simulink model "OFDM"  (R2021a)
settings: Solver=VariableStepAuto  StartTime=0.0  StopTime=1000.0  RelTol=1e-3
InitFcn:
  | clear
  | %frequency
  | Fs = 20e6;
  | M =16;
  | 
  | fD=1;
  | Td=[0, 200, 300, 1300, 2700]*1e-09;
  | Pd=[0, -0.9, -3.9, -7.8, -13.9];
undefined symbols (not defined in the file or in its folder): doppler
libraries: commutil2 x2, dspxfrm3 x2, commdigbbndam3 x2, commrandsrc3 x1, commsink2 x1, commchan3 x1
settings Model: Creator=AJ  LastModifiedBy=AJ
settings SFSimCC: MATLABDynamicMemAllocThreshold=2147483647

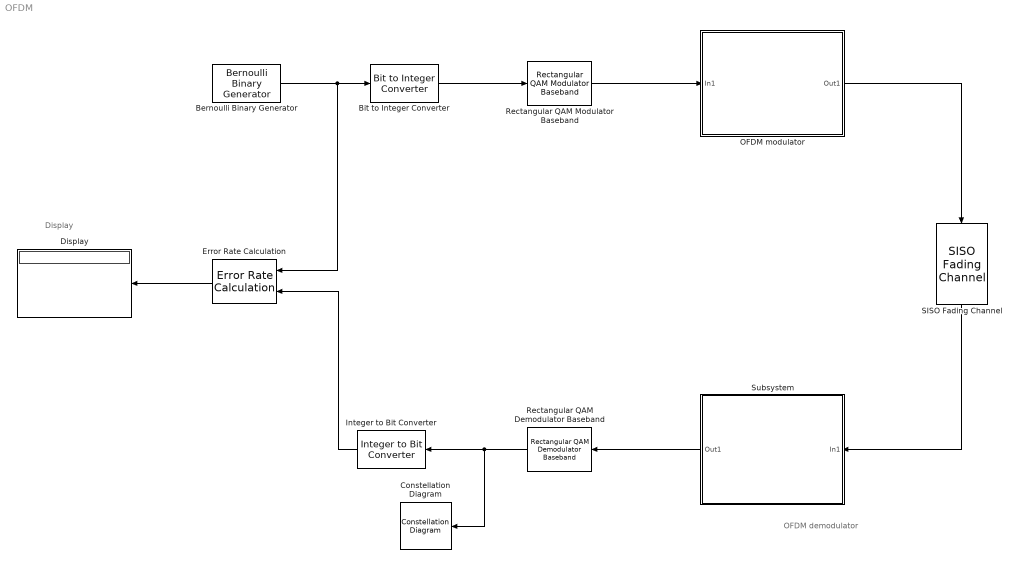
== system OFDM ==
  note: Display
  note: OFDM demodulator
  Bernoulli Binary Generator : commrandsrc3/Bernoulli Binary Generator  ProbabilityOfZero=0.5  SeedSource=Parameter  Seed=61  SampleTime=1/Fs  SamplesPerFrame=52*log2(M)  OutputDataType=double  SimulateUsing=Interpreted execution
  Bit to Integer Converter : commutil2/Bit to Integer Converter  nbits=log2(M)  bitOrder=MSB first  signedOutputValues=Unsigned  outDtype=Inherit via internal rule  outDtypeSigned=Inherit via internal rule
  Constellation Diagram : ConstellationDiagram
  Display : Display
  Error Rate Calculation : commsink2/Error Rate Calculation  N=0  st_delay=0  cp_mode=Entire frame  subframe=[]  PMode=Port  WsName=ErrorVec  RsMode2=off  stop=on  numErr=100  maxBits=1e6
  Integer to Bit Converter : commutil2/Integer to Bit Converter  nbits=log2(M)  signedInputValues=Unsigned  bitOrder=MSB first  outDtype=Inherit via internal rule
  OFDM modulator : Subsystem
  Rectangular QAM Demodulator Baseband : commdigbbndam3/Rectangular QAM Demodulator Baseband  M=M  OutType=Integer  DecType=Hard decision  VarSource=Dialog  Variance=1  Dec=Gray  Mapping=[0:15]  PowType=Average Power  MinDist=2  AvgPow=1  PeakPow=1  Ph=0  outDtype1=Inherit via internal rule  outDtype2=Inherit via internal rule  derotateFactorWordLen=16  derotateFactorDataTypeStr=Inherit: Same word length as input  derotateFactorLastDataTypeStr=Inherit: Same word length as input  denormFactorWordLen=16  denormFactorDataTypeStr=Inherit: Same word length as input  denormFactorLastDataTypeStr=Inherit: Same word length as input  prodOutWordLen=32  prodOutOverflowMode=Wrap  prodOutRoundingMode=Floor  prodOutOvFlMode=off  prodOutOvFlModeLastStrValue=off  sumWordLen=32
  Rectangular QAM Modulator Baseband : commdigbbndam3/Rectangular QAM Modulator Baseband  M=M  InType=Integer  Enc=Gray  Mapping=[0:15]  PowType=Average Power  MinDist=2  AvgPow=1  PeakPow=1  Ph=0  outDtype=double  outWordLen=16  outUDDataType=sfix(16)  outFracLenMode=Best precision  outFracLen=15  outDataTypeStr=double  outLastDataTypeStr=double
  SISO Fading Channel : commchan3/SISO Fading Channel  InheritSampleRate=on  SampleRate=1  PathDelays=Td  AveragePathGains=Pd  NormalizePathGains=on  FadingDistribution=Rayleigh  KFactor=3  DirectPathDopplerShift=0  DirectPathInitialPhase=0  MaximumDopplerShift=fD  DopplerSpectrum=doppler('Jakes')  RandomStream=mt19937ar with seed  Seed=61  PathGainsOutputPort=off  ChannelFilterDelayOutputPort=off  SimulateUsing=Interpreted execution  Visualization=Off  PathsForDopplerDisplay=1  SamplesToDisplay=25%
  Subsystem : Subsystem
  wires:
  Error Rate Calculation/1 -> Display/1
  Bit to Integer Converter/1 -> Rectangular QAM Modulator Baseband/1
  Rectangular QAM Demodulator Baseband/1 -> Constellation Diagram/1, Integer to Bit Converter/1
  Integer to Bit Converter/1 -> Error Rate Calculation/2
  Bernoulli Binary Generator/1 -> Error Rate Calculation/1, Bit to Integer Converter/1
  OFDM modulator/1(Out1) -> SISO Fading Channel/1
  SISO Fading Channel/1 -> Subsystem/1(In1)
  Rectangular QAM Modulator Baseband/1 -> OFDM modulator/1(In1)
  Subsystem/1(Out1) -> Rectangular QAM Demodulator Baseband/1

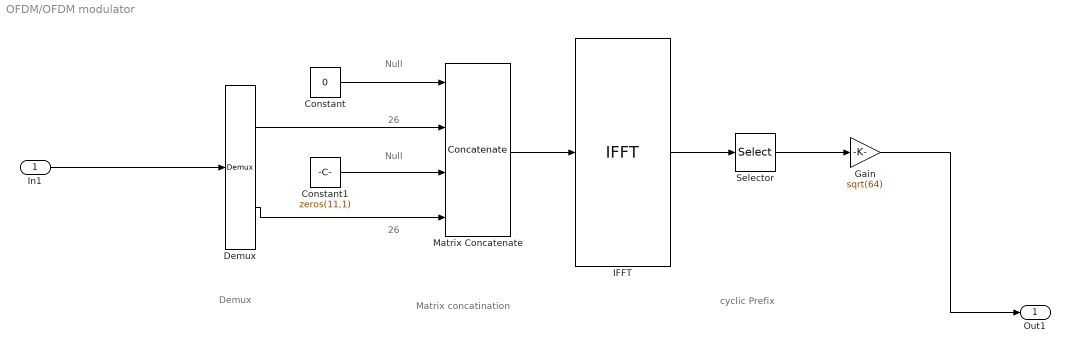
== system OFDM/OFDM modulator ==
  note: Null
  note: 26
  note: 26
  note: cyclic Prefix
  note: Matrix concatination
  note: Demux
  note: Null
  In1 : Inport
  Constant : Constant  Value=0
  Constant1 : Constant  Value=zeros(11,1)
  Demux : Demux  Outputs=[26,26]
  Gain : Gain  Gain=sqrt(64)
  IFFT : dspxfrm3/IFFT  FFTImplementation=Auto  CompMethod=Table lookup  TableOpt=NEW  TableOptActive=Speed  BitRevOrder=off  cs_in=off  Normalize=on  InheritFFTLength=off  FFTLength=64  WrapInput=on  mode=Complex  outSamplingMode=Sample based  roundingMode=Floor  overflowMode=off  firstCoeffDataTypeStr=Inherit: Same word length as input  firstCoeffLastDataTypeStr=Inherit: Same word length as input  outputMin=[]  outputMax=[]
  Matrix Concatenate : Concatenate  NumInputs=4  Mode=Multidimensional array
  Selector : Selector  InputPortWidth=64  IndexOptions=Index vector (dialog)  Indices=[49:64, 1: 64]  OutputSizes=1
  Out1 : Outport
  wires:
  Constant1/1 -> Matrix Concatenate/3
  IFFT/1 -> Selector/1
  Selector/1 -> Gain/1
  Demux/1 -> Matrix Concatenate/2
  Constant/1 -> Matrix Concatenate/1
  Gain/1 -> Out1/1
  Matrix Concatenate/1 -> IFFT/1
  Demux/2 -> Matrix Concatenate/4
  In1/1 -> Demux/1

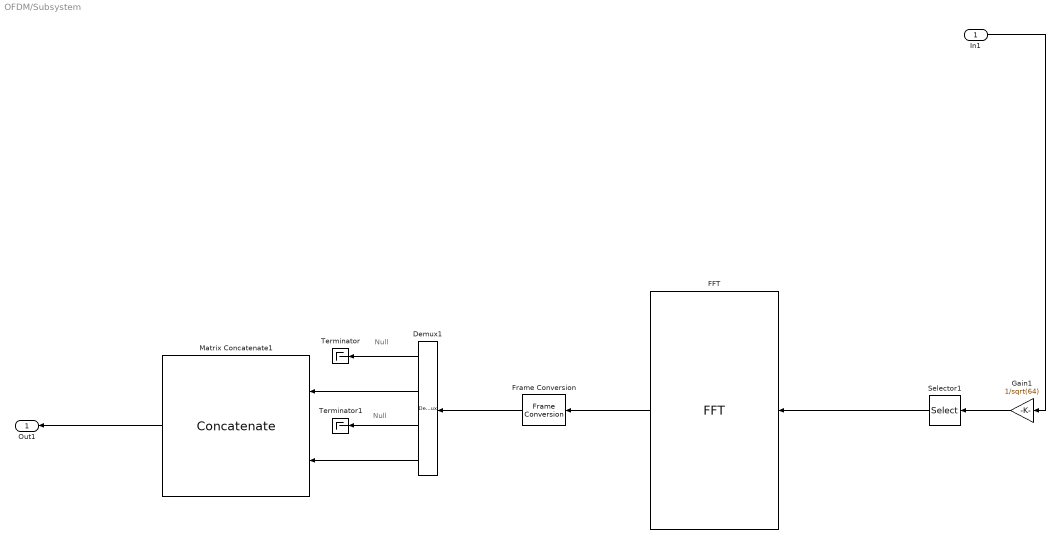
== system OFDM/Subsystem ==
  note: Null
  note: Null
  In1 : Inport
  Demux1 : Demux  Outputs=[1,26,11,26]
  FFT : dspxfrm3/FFT  FFTImplementation=Auto  CompMethod=Table lookup  TableOpt=NEW  TableOptActive=Speed  BitRevOrder=off  Normalize=off  InheritFFTLength=on  FFTLength=64  WrapInput=on  roundingMode=Floor  overflowMode=off  firstCoeffDataTypeStr=Inherit: Same word length as input  firstCoeffLastDataTypeStr=Inherit: Same word length as input  outputMin=[]  outputMax=[]
  Frame Conversion : FrameConversion
  Gain1 : Gain  Gain=1/sqrt(64)
  Matrix Concatenate1 : Concatenate  Mode=Multidimensional array
  Selector1 : Selector  InputPortWidth=80  IndexOptions=Index vector (dialog)  Indices=[17:80]  OutputSizes=1
  Terminator : Terminator
  Terminator1 : Terminator
  Out1 : Outport
  wires:
  In1/1 -> Gain1/1
  Selector1/1 -> FFT/1
  Gain1/1 -> Selector1/1
  FFT/1 -> Frame Conversion/1
  Matrix Concatenate1/1 -> Out1/1
  Frame Conversion/1 -> Demux1/1
  Demux1/1 -> Terminator/1
  Demux1/3 -> Terminator1/1
  Demux1/2 -> Matrix Concatenate1/1
  Demux1/4 -> Matrix Concatenate1/2
